simulink model "demoUSBserial"  (R2016a)
settings: Solver=FixedStepAuto  StartTime=0.0  StopTime=10.0  RelTol=1e-3
libraries: frdmKL25Z x2, frdmkl25zlib x1
settings Model: ExtModeTrigDuration=5  Creator=user  LastModifiedBy=user
settings OptimizationCC: OptimizeModelRefInitCode=on  LifeSpan=1  MaxStackSize=64
settings HardwareCC: ProdBitPerPointer=32  ProdLargestAtomicInteger=Long  ProdLargestAtomicFloat=Double  ProdWordSize=32  ProdHWDeviceType=ARM Compatible->ARM Cortex
settings RTWCC: SystemTargetFile=ert.tlc  HardwareBoard=Freescale FRDM-KL25Z  TemplateMakefile=ert_default_tmf  GenerateReport=on  Toolchain=GNU Tools for ARM Embedded Processors  IncludeHyperlinkInReport=on  LaunchReport=on  GenerateTraceInfo=on  GenerateTraceReport=on  GenerateTraceReportSl=on  GenerateTraceReportSf=on  GenerateTraceReportEml=on
settings CodeAppCC: ForceParamTrailComments=on  IgnoreCustomStorageClasses=off  OperatorAnnotations=on  SimulinkDataObjDesc=on  SFDataObjDesc=on  MATLABFcnDesc=on  InsertBlockDesc=on  MATLABSourceComments=on

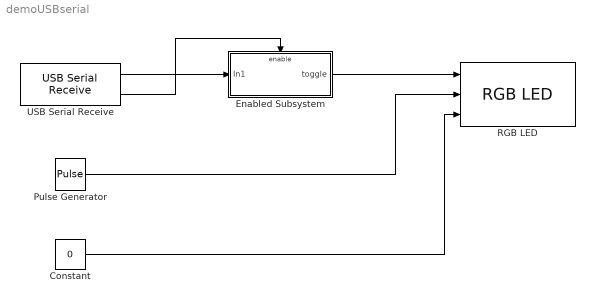
== system demoUSBserial ==
  Constant : Constant  Value=0
  Enabled Subsystem : Subsystem  TreatAsAtomicUnit=on
  Pulse Generator : DiscretePulseGenerator  Amplitude=100
  RGB LED : frdmkl25zlib/RGB LED
  USB Serial Receive : frdmKL25Z/USB Serial Receive
  wires:
  USB Serial Receive/1 -> Enabled Subsystem/1(In1)
  USB Serial Receive/2 -> Enabled Subsystem/Enable
  Enabled Subsystem/1(toggle) -> RGB LED/1
  Pulse Generator/1 -> RGB LED/2
  Constant/1 -> RGB LED/3

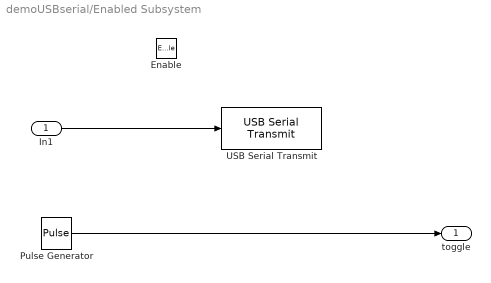
== system demoUSBserial/Enabled Subsystem ==
  In1 : Inport
  Enable : EnablePort
  Pulse Generator : DiscretePulseGenerator  Amplitude=100  SampleTime=-1
  USB Serial Transmit : frdmKL25Z/USB Serial Transmit
  toggle : Outport
  wires:
  In1/1 -> USB Serial Transmit/1
  Pulse Generator/1 -> toggle/1
